simulink library "AdaptiveLib"  (R2022b)
settings: Solver=VariableStepAuto  StartTime=0.0  StopTime=10.0  RelTol=1e-3
settings Model: Creator=tbritton  LastModifiedBy=macheson
settings SolverCC: AlgebraicLoopSolver=TrustRegion
settings DebuggingCC: UnconnectedInputMsg=warning  UnconnectedOutputMsg=warning  UnconnectedLineMsg=warning  SFMachineParentedDataDiag=warning
settings ModelReferenceCC: EnableRefExpFcnMdlSchedulingChecks=on
settings RTWCC: DLArmComputeVersion=19.05

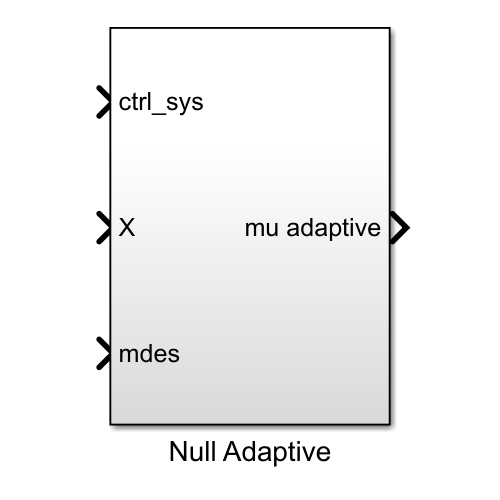
[thumbnail: Simulink's stored preview of the top-level diagram]
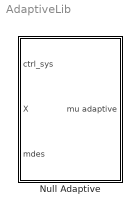
== system AdaptiveLib ==
  Null Adaptive : Subsystem

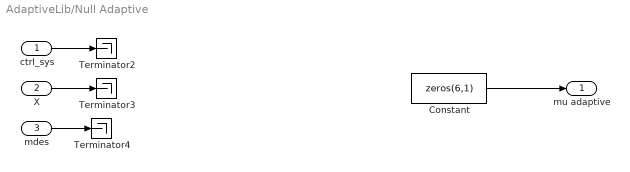
== system AdaptiveLib/Null Adaptive ==
  ctrl_sys : Inport
  X : Inport  Port=2
  mdes : Inport  Port=3
  Constant : Constant  Value=zeros(6,1)
  Terminator2 : Terminator
  Terminator3 : Terminator
  Terminator4 : Terminator
  mu adaptive : Outport
  wires:
  Constant/1 -> mu adaptive/1
  ctrl_sys/1 -> Terminator2/1
  X/1 -> Terminator3/1
  mdes/1 -> Terminator4/1
